simulink model "EPT"  (R2019b)
settings: Solver=FixedStepDiscrete  StartTime=0.0  StopTime=5  FixedStep=0.005  RelTol=1e-3  EnableMultiTasking=on
PreLoadFcn:
  | try, model_open; catch, disp('Error occurred while executing model pre-load callback: model_open.m'); disp('Please assure that the MATLAB working directory is set to the model directory before opening.'); end
InitFcn:
  | try, model_open; catch, end
undefined symbols (not defined in the file or in its folder): Bridge, GCM, H, ln, raptor_get_param_eval, raptor_get_safe_string, raptor_xcp_function
libraries: Raptor_lib x2810, simulink x374, hdlsllib x19
(part 4 of 45)

== system EPT/Foreground_TimeBase_5ms/CHG//DCHG_PW_Control/Maximum allowable torque ==
  note: P(KW)= Torque*rpm/9549.297
  Idchg_con : Inport
  Abs : Abs
  Abs1 : Abs
  Compare To Constant : simulink/Logic and Bit Operations/Compare To Constant  relop=<=  const=5  OutDataTypeStr=boolean
  Constant : Constant
  Data Type Conversion : DataTypeConversion
  Data Type Conversion1 : DataTypeConversion
  Data Type Conversion2 : DataTypeConversion
  Delay : Delay  DelayLength=1  InitialCondition=0
  Divide : Product  Inputs=*/
  Gain1 : Gain  Gain=0.01
  Gain2 : Gain  Gain=9.54805
  Min : MinMax  Inputs=2
  Product : Product  Inputs=3
  Product1 : Product
  Saturation : Saturate  UpperLimit=150  LowerLimit=0
  Saturation Dynamic1 : simulink/Discontinuities/Saturation Dynamic  OutMin=[]  OutMax=[]  OutDataTypeStr=Inherit: Same as second input  OutDataType=fixdt(1, 16)  OutScaling=2^-10  DoSatur=off
  Subtract : Sum  Inputs=+-
  Switch : Switch  Criteria=u2 > Threshold
  raptor_adjustment1 : Raptor_lib/Data Storage/raptor_adjustment  paramName='Cal_Eff_Min'  nameSource=Parameter  initValue=0  dataType=double  storage=Calibration  calDispType=Number  calEnum={'False', 'True'}  calGain=1.0  calOffset=0.0  calMax=inf  calMin=-inf  calFormat='-1'  calUnit=''  calHelp=''  calAccess=1  calFunction=raptor_xcp_function(gcb)  calDispHeaders=off  calColHeaders={'Col1' 'Col2' 'Col3'}  calRowHeaders={'Row1' 'Row2' 'Row3'}
      settings: SourceProductName=Raptor
  raptor_adjustment2 : Raptor_lib/Data Storage/raptor_adjustment  paramName='Vehicle_system_power'  nameSource=Parameter  initValue=5000  dataType=double  storage=Calibration  calDispType=Number  calEnum={'False', 'True'}  calGain=1.0  calOffset=0.0  calMax=inf  calMin=-inf  calFormat='-1'  calUnit=''  calHelp=''  calAccess=1  calFunction=raptor_xcp_function(gcb)  calDispHeaders=off  calColHeaders={'Col1' 'Col2' 'Col3'}  calRowHeaders={'Row1' 'Row2' 'Row3'}
      settings: SourceProductName=Raptor
  raptor_adjustment3 : Raptor_lib/Data Storage/raptor_adjustment  paramName='Cal_Eff_Max'  nameSource=Parameter  initValue=100  dataType=double  storage=Calibration  calDispType=Number  calEnum={'False', 'True'}  calGain=1.0  calOffset=0.0  calMax=inf  calMin=-inf  calFormat='-1'  calUnit=''  calHelp=''  calAccess=1  calFunction=raptor_xcp_function(gcb)  calDispHeaders=off  calColHeaders={'Col1' 'Col2' 'Col3'}  calRowHeaders={'Row1' 'Row2' 'Row3'}
      settings: SourceProductName=Raptor
  raptor_data_read1 : Raptor_lib/Data Storage/raptor_data_read  dataName='EPT_BPOBU_VOLT'  dataShape=Scalar  idxSource=Input  idxRow=1  idxCol=1
      settings: SourceProductName=Raptor
  raptor_data_read2 : Raptor_lib/Data Storage/raptor_data_read  dataName='Read_Motor_Speed'  dataShape=Scalar  idxSource=Input  idxRow=1  idxCol=1
      settings: SourceProductName=Raptor
  raptor_data_read3 : Raptor_lib/Data Storage/raptor_data_read  dataName='Read_Motor_Temp'  dataShape=Scalar  idxSource=Input  idxRow=1  idxCol=1
      settings: SourceProductName=Raptor
  raptor_data_read4 : Raptor_lib/Data Storage/raptor_data_read  dataName='Read_Controller_Temp'  dataShape=Scalar  idxSource=Input  idxRow=1  idxCol=1
      settings: SourceProductName=Raptor
  raptor_data_write : Raptor_lib/Data Storage/raptor_data_write  dataName='EPT_MAX_DRV_TRQ'  dataShape=Scalar  idxSource=Input Port  idxRow=1  idxCol=1
      settings: SourceProductName=Raptor
  raptor_measurement1 : Raptor_lib/Data Storage/raptor_measurement  paramName='efficiency'  nameSource=Parameter  calDispType=Number  calEnum={'False', 'True'}  calGain=1.0  calOffset=0.0  calMax=inf  calMin=-inf  calFormat='-1'  calUnit=''  calHelp=''  calAccess=1  calFunction=raptor_xcp_function(gcb)  calVisible=on
      settings: SourceProductName=Raptor
  raptor_measurement3 : Raptor_lib/Data Storage/raptor_measurement  paramName='tqMax_con'  nameSource=Parameter  calDispType=Number  calEnum={'False', 'True'}  calGain=1.0  calOffset=0.0  calMax=inf  calMin=-inf  calFormat='-1'  calUnit=''  calHelp=''  calAccess=1  calFunction=raptor_xcp_function(gcb)  calVisible=on
      settings: SourceProductName=Raptor
  raptor_table_1d1 : Raptor_lib/Table Lookup/raptor_table_1d  dataName='Tcontroller2MaxTq_Ft'  initValue=[1 1 0]  dataType=double  storage=Calibration  initValueX=[0 60 80]  dataTypeXY=double  storageXY=Calibration  calVisible=on  showTable=on  calGain=1.0  calOffset=0.0  calMax=Inf  calMin=-Inf  calFormat='-1'  calUnit=''  calHelp=''  showBreakpoint=on  dataNameX=[]  calGainX=1.0  calOffsetX=0.0  calMaxX=Inf  calMinX=-Inf  calFormatX='-1'  calUnitX=''  calHelpX=''  calAccess=1  calFunction=raptor_xcp_function(gcb)  measureEnable=off  mName=[raptor_get_param_eval(gcb,'dataName'), '_Output']
      settings: SourceProductName=Raptor
  raptor_table_1d2 : Raptor_lib/Table Lookup/raptor_table_1d  dataName='Tmotor2MaxTq_Ft'  initValue=[1 1 0]  dataType=double  storage=Calibration  initValueX=[0 100 120]  dataTypeXY=double  storageXY=Calibration  calVisible=on  showTable=on  calGain=1.0  calOffset=0.0  calMax=Inf  calMin=-Inf  calFormat='-1'  calUnit=''  calHelp=''  showBreakpoint=on  dataNameX=[]  calGainX=1.0  calOffsetX=0.0  calMaxX=Inf  calMinX=-Inf  calFormatX='-1'  calUnitX=''  calHelpX=''  calAccess=1  calFunction=raptor_xcp_function(gcb)  measureEnable=off  mName=[raptor_get_param_eval(gcb,'dataName'), '_Output']
      settings: SourceProductName=Raptor
  raptor_table_2d : Raptor_lib/Table Lookup/raptor_table_2d  dataName='Efficiency'  initValue=|  dataType=double  storage=Calibration  initValueX="[0\t300\t600\t1200\t1800\t2400\t3000\t3600\t4200\t4800\t5400\t6000]"  initValueY="[0\t7.5\t15\t30\t45\t60\t75\t90\t105\t120\t135\t150]"  dataTypeXY=double  storageXY=Calibration  calVisible=on  showTable=off  calGain=1.0  calOffset=0.0  calMax=Inf  calMin=-Inf  calFormat='-1'  calUnit=''  calHelp=''  showBreakpointX=off  dataNameX=[]  calGainX=1.0  calOffsetX=0.0  calMaxX=Inf  calMinX=-Inf  calFormatX='-1'  calUnitX=''  calHelpX=''  showBreakpointY=off  dataNameY=[]  calGainY=1.0  calOffsetY=0.0  calMaxY=Inf  calMinY=-Inf  calFormatY='-1'  calUnitY=''  calHelpY=''  calAccess=1  calFunction=raptor_xcp_function(gcb)  measureEnable=off  mName=[raptor_get_param_eval(gcb,'dataName'), '_Output']
      | [50	50	50	50	50	50	50	50	50	50	50	50;
      | 55	60	62.5	65	70	72.5	75	77.5	77.5	75	72.5	70;
      | 57.5	62.5	65	70	77.5	80	80	82.5	82.5	80	77.5	75;
      | 57.5	65	67.5	72.5	80	82.5	85	85	85	85	85	82.5;
      | 60	67.5	70	80	85	85	87.5	87.5	87.5	87.5	87.5	85;
      | 60	67.5	72.5	82.5	87.5	87.5	90	90	90	87.5	85	82.5;
      | 62.5	70	75	82.5	87.5	90	90	87.5	85	82.5	82.5	80;
      | 62.5	72.5	77.5	85	90	90	87.5	85	82.5	80	80	77.5;
      | 65	72.5	77.5	85	90	90	85	82.5	80	77.5	80	75;
      | 65	72.5	75	82.5	90	87.5	82.5	80	80	75	77.5	72.5;
      | 67.5	70	75	82.5	87.5	85	82.5	80	77.5	75	75	70;
      | 67.5	70	72.5	80	85	82.5	77.5	75	77.5	72.5	75	70;]
      settings: SourceProductName=Raptor
  wires:
  Gain2/1 -> Divide/1
  Idchg_con/1 -> Abs/1
  Subtract/1 -> Gain2/1
  raptor_adjustment2/1 -> Subtract/2
  Switch/1 -> Divide/2
  Product/1 -> Subtract/1
  Abs/1 -> Product/3
  raptor_data_read1/1 -> Product/2
  raptor_data_read2/1 -> Abs1/1
  Compare To Constant/1 -> Switch/2
  Constant/1 -> Switch/1
  Saturation Dynamic1/1 -> raptor_measurement1/1, Gain1/1
  Gain1/1 -> Product/1
  Abs1/1 -> Data Type Conversion/1
  Data Type Conversion/1 -> raptor_table_2d/2, Switch/3, Compare To Constant/1
  Divide/1 -> Saturation/1
  Delay/1 -> raptor_table_2d/1
  Data Type Conversion1/1 -> raptor_data_write/1
  raptor_data_read3/1 -> raptor_table_1d2/1
  Min/1 -> Product1/1
  Saturation/1 -> Product1/2, Delay/1
  Product1/1 -> Data Type Conversion1/1, raptor_measurement3/1
  raptor_table_2d/1 -> Saturation Dynamic1/2
  raptor_adjustment3/1 -> Saturation Dynamic1/1
  raptor_adjustment1/1 -> Saturation Dynamic1/3
  raptor_data_read4/1 -> Data Type Conversion2/1
  raptor_table_1d1/1 -> Min/1
  raptor_table_1d2/1 -> Min/2
  Data Type Conversion2/1 -> raptor_table_1d1/1

== system EPT/Foreground_TimeBase_5ms/CHG//DCHG_PW_Control/PWCU PW Requirement ==

== system EPT/Foreground_TimeBase_5ms/CHG//DCHG_PW_Control/SWU Power Divider ==
  PWCU : Subsystem

== system EPT/Foreground_TimeBase_5ms/Delay/CycleTrigger ==
  In1 : Inport
  In2 : Inport  Port=2
  Add : Sum
  Add1 : Sum
  Add2 : Sum  Inputs=+-
  Constant1 : Constant
  Constant2 : Constant  Value=0
  Constant3 : Constant
  Data Type Conversion1 : DataTypeConversion
  Data Type Conversion2 : DataTypeConversion
  Display : Display
  Relational Operator1 : RelationalOperator  OutDataTypeStr=boolean  RndMeth=Simplest
  Saturation : Saturate  UpperLimit=inf  LowerLimit=2
  Scope : Scope
  Scope1 : Scope
  Scope2 : Scope
  Switch : Switch  Threshold=1
  Unit Delay : UnitDelay  SampleTime=-1  HasFrameUpgradeWarning=on
  Unit Delay1 : UnitDelay  SampleTime=-1  HasFrameUpgradeWarning=on
  Trigger : Outport  VectorParamsAs1DForOutWhenUnconnected=off
  wires:
  Saturation/1 -> Add2/1
  Add/1 -> Switch/1
  In1/1 -> Data Type Conversion2/1
  Unit Delay/1 -> Add/1
  Switch/1 -> Relational Operator1/1, Scope1/1, Unit Delay/1
  Add1/1 -> Scope/1, Unit Delay1/1, Display/1
  Unit Delay1/1 -> Add1/1
  Constant1/1 -> Add1/2
  Relational Operator1/1 -> Scope2/1, Trigger/1
  Data Type Conversion1/1 -> Relational Operator1/2
  Constant2/1 -> Switch/3
  Data Type Conversion2/1 -> Add/2, Switch/2
  Add2/1 -> Data Type Conversion1/1
  In2/1 -> Saturation/1
  Constant3/1 -> Add2/2

== system EPT/Foreground_TimeBase_5ms/E//W /BP-OBU_E//W ==
  BP-OBU_E/W : Subsystem
  Delay : Subsystem
  Latch : Subsystem
  Logical Operator1 : Logic  Inputs=3  AllPortsSameDT=off  OutDataTypeStr=boolean
  NOT : Logic  Operator=NOT  IconShape=distinctive  AllPortsSameDT=off  OutDataTypeStr=boolean
  NOT1 : Logic  Operator=NOT  IconShape=distinctive  AllPortsSameDT=off  OutDataTypeStr=boolean
  NOT2 : Logic  Operator=NOT  IconShape=distinctive  AllPortsSameDT=off  OutDataTypeStr=boolean
  raptor_adjustment : Raptor_lib/Data Storage/raptor_adjustment  paramName='Cal_BPOBU_EW_Check_TimeCount'  nameSource=Parameter  initValue=400  dataType=double  storage=Calibration  calDispType=Number  calEnum={'False', 'True'}  calGain=1.0  calOffset=0.0  calMax=inf  calMin=-inf  calFormat='-1'  calUnit=''  calHelp=''  calAccess=1  calFunction=raptor_xcp_function(gcb)  calDispHeaders=off  calColHeaders={'Col1' 'Col2' 'Col3'}  calRowHeaders={'Row1' 'Row2' 'Row3'}
      settings: SourceProductName=Raptor
  raptor_data_read1 : Raptor_lib/Data Storage/raptor_data_read  dataName='CMU_Ready'  dataShape=Scalar  idxSource=Input  idxRow=1  idxCol=1
      settings: SourceProductName=Raptor
  raptor_data_read19 : Raptor_lib/Data Storage/raptor_data_read  dataName='CAN_Fault_CMU1'  dataShape=Scalar  idxSource=Input  idxRow=1  idxCol=1
      settings: SourceProductName=Raptor
  raptor_data_read20 : Raptor_lib/Data Storage/raptor_data_read  dataName='CAN_Fault_CMU2'  dataShape=Scalar  idxSource=Input  idxRow=1  idxCol=1
      settings: SourceProductName=Raptor
  wires:
  Delay/1(Output) -> Latch/1(Latch)
  raptor_data_read19/1 -> NOT/1
  raptor_data_read20/1 -> NOT1/1
  raptor_adjustment/1 -> Delay/2(TimeCount)
  Logical Operator1/1 -> NOT2/1, Delay/1(Condition)
  NOT/1 -> Logical Operator1/2
  NOT2/1 -> Latch/2(Reset)
  NOT1/1 -> Logical Operator1/3
  Latch/1(Output) -> BP-OBU_E/W/1("CMU_Work ")
  raptor_data_read1/1 -> Logical Operator1/1

== system EPT/Foreground_TimeBase_5ms/E//W /CAN_E//W ==
  CAN_Abnormal : Subsystem
  CAN_Fault : Subsystem

== system EPT/Foreground_TimeBase_5ms/E//W /E//W_Process ==
  CAN_Fault : Subsystem
  Data Type Conversion1 : DataTypeConversion
  ECHS_Fault : Subsystem
  Logical Operator : Logic  Operator=OR  Inputs=6  AllPortsSameDT=off  OutDataTypeStr=boolean
  OBU_Fault : Subsystem
  Switch3 : Switch  Threshold=1
  raptor_adjustment1 : Raptor_lib/Data Storage/raptor_adjustment  paramName='Cal_Alarm_Manual'  nameSource=Parameter  initValue=0.00  dataType=boolean  storage=Calibration  calDispType=Number  calEnum={'False', 'True'}  calGain=1.0  calOffset=0.0  calMax=inf  calMin=-inf  calFormat='-1'  calUnit=''  calHelp=''  calAccess=1  calFunction=raptor_xcp_function(gcb)  calDispHeaders=off  calColHeaders={'Col1' 'Col2' 'Col3'}  calRowHeaders={'Row1' 'Row2' 'Row3'}
      settings: SourceProductName=Raptor
  raptor_adjustment2 : Raptor_lib/Data Storage/raptor_adjustment  paramName='Cal_Alarm_Manual_EN'  nameSource=Parameter  initValue=0.00  dataType=boolean  storage=Calibration  calDispType=Number  calEnum={'False', 'True'}  calGain=1.0  calOffset=0.0  calMax=inf  calMin=-inf  calFormat='-1'  calUnit=''  calHelp=''  calAccess=1  calFunction=raptor_xcp_function(gcb)  calDispHeaders=off  calColHeaders={'Col1' 'Col2' 'Col3'}  calRowHeaders={'Row1' 'Row2' 'Row3'}
      settings: SourceProductName=Raptor
  raptor_data_def6 : Raptor_lib/Data Storage/raptor_data_def  dataName='EPT_EW_STA'  initValue=0  dataType=boolean  storage=Volatile (RAM)  calVisible=on  calType=Measurement  calDispType=Number  calEnum={'False', 'True'}  calGain=1.0  calOffset=0  calMin=-inf  calMax=inf  calFormat='-1'  calUnit=''  calHelp=''  calAccess=1  calFunction=raptor_xcp_function(gcb)  calDispHeaders=off  calColHeaders={'Col1' 'Col2' 'Col3'}  calRowHeaders={'Row1' 'Row2' 'Row3'}
      settings: SourceProductName=Raptor
  raptor_data_write4 : Raptor_lib/Data Storage/raptor_data_write  dataName='EPT_EW_STA'  dataShape=Scalar  idxSource=Input Port  idxRow=1  idxCol=1
      settings: SourceProductName=Raptor
  wires:
  raptor_adjustment2/1 -> Switch3/2
  Switch3/1 -> Data Type Conversion1/1
  raptor_adjustment1/1 -> Switch3/1
  Data Type Conversion1/1 -> raptor_data_write4/1
  CAN_Fault/1(Fault) -> Logical Operator/1
  Logical Operator/1 -> Switch3/3
  ECHS_Fault/1(Fault) -> Logical Operator/2
  OBU_Fault/1(G1_Fault) -> Logical Operator/3
  OBU_Fault/2(G2_Fault) -> Logical Operator/4
  OBU_Fault/3(G3_Fault) -> Logical Operator/5
  OBU_Fault/4(G4_Fault) -> Logical Operator/6

== system EPT/Foreground_TimeBase_5ms/OBP_Temp_Detection/ADC2Degree ==
  Trigger : TriggerPort  VariantControl=Variant  PortDimensions=1
  Data Type Conversion : DataTypeConversion
  Demux : Demux
  Gain : Gain  Gain=1/4
  MinMax : MinMax  Function=max
  MinMax1 : MinMax
  Mux : Mux
  Mux1 : Mux
  Sum of Elements : Sum  Inputs=+
  raptor_data_def1 : Raptor_lib/Data Storage/raptor_data_def  dataName='Temp_1'  initValue=0  dataType=double  storage=Volatile (RAM)  calVisible=on  calType=Measurement  calDispType=Number  calEnum={'False', 'True'}  calGain=1.0  calOffset=0  calMin=-inf  calMax=inf  calFormat='-1'  calUnit=''  calHelp=''  calAccess=1  calFunction=raptor_xcp_function(gcb)  calDispHeaders=off  calColHeaders={'Col1' 'Col2' 'Col3'}  calRowHeaders={'Row1' 'Row2' 'Row3'}
      settings: SourceProductName=Raptor
  raptor_data_def2 : Raptor_lib/Data Storage/raptor_data_def  dataName='Temp_2'  initValue=0  dataType=double  storage=Volatile (RAM)  calVisible=on  calType=Measurement  calDispType=Number  calEnum={'False', 'True'}  calGain=1.0  calOffset=0  calMin=-inf  calMax=inf  calFormat='-1'  calUnit=''  calHelp=''  calAccess=1  calFunction=raptor_xcp_function(gcb)  calDispHeaders=off  calColHeaders={'Col1' 'Col2' 'Col3'}  calRowHeaders={'Row1' 'Row2' 'Row3'}
      settings: SourceProductName=Raptor
  raptor_data_def3 : Raptor_lib/Data Storage/raptor_data_def  dataName='Temp_3'  initValue=0  dataType=double  storage=Volatile (RAM)  calVisible=on  calType=Measurement  calDispType=Number  calEnum={'False', 'True'}  calGain=1.0  calOffset=0  calMin=-inf  calMax=inf  calFormat='-1'  calUnit=''  calHelp=''  calAccess=1  calFunction=raptor_xcp_function(gcb)  calDispHeaders=off  calColHeaders={'Col1' 'Col2' 'Col3'}  calRowHeaders={'Row1' 'Row2' 'Row3'}
      settings: SourceProductName=Raptor
  raptor_data_def4 : Raptor_lib/Data Storage/raptor_data_def  dataName='Temp_4'  initValue=0  dataType=double  storage=Volatile (RAM)  calVisible=on  calType=Measurement  calDispType=Number  calEnum={'False', 'True'}  calGain=1.0  calOffset=0  calMin=-inf  calMax=inf  calFormat='-1'  calUnit=''  calHelp=''  calAccess=1  calFunction=raptor_xcp_function(gcb)  calDispHeaders=off  calColHeaders={'Col1' 'Col2' 'Col3'}  calRowHeaders={'Row1' 'Row2' 'Row3'}
      settings: SourceProductName=Raptor
  raptor_data_def5 : Raptor_lib/Data Storage/raptor_data_def  dataName='BP_OBU_Tbp_Down'  initValue=0  dataType=double  storage=Volatile (RAM)  calVisible=on  calType=Measurement  calDispType=Number  calEnum={'False', 'True'}  calGain=1.0  calOffset=0  calMin=-inf  calMax=inf  calFormat='-1'  calUnit=''  calHelp=''  calAccess=1  calFunction=raptor_xcp_function(gcb)  calDispHeaders=off  calColHeaders={'Col1' 'Col2' 'Col3'}  calRowHeaders={'Row1' 'Row2' 'Row3'}
      settings: SourceProductName=Raptor
  raptor_data_def6 : Raptor_lib/Data Storage/raptor_data_def  dataName='BP_OBU_Tbp_Up'  initValue=0  dataType=double  storage=Volatile (RAM)  calVisible=on  calType=Measurement  calDispType=Number  calEnum={'False', 'True'}  calGain=1.0  calOffset=0  calMin=-inf  calMax=inf  calFormat='-1'  calUnit=''  calHelp=''  calAccess=1  calFunction=raptor_xcp_function(gcb)  calDispHeaders=off  calColHeaders={'Col1' 'Col2' 'Col3'}  calRowHeaders={'Row1' 'Row2' 'Row3'}
      settings: SourceProductName=Raptor
  raptor_data_def7 : Raptor_lib/Data Storage/raptor_data_def  dataName='BP_OBU_Tair_In'  initValue=0  dataType=double  storage=Volatile (RAM)  calVisible=on  calType=Measurement  calDispType=Number  calEnum={'False', 'True'}  calGain=1.0  calOffset=0  calMin=-inf  calMax=inf  calFormat='-1'  calUnit=''  calHelp=''  calAccess=1  calFunction=raptor_xcp_function(gcb)  calDispHeaders=off  calColHeaders={'Col1' 'Col2' 'Col3'}  calRowHeaders={'Row1' 'Row2' 'Row3'}
      settings: SourceProductName=Raptor
  raptor_data_def8 : Raptor_lib/Data Storage/raptor_data_def  dataName='BP_OBU_Tair_Out'  initValue=0  dataType=double  storage=Volatile (RAM)  calVisible=on  calType=Measurement  calDispType=Number  calEnum={'False', 'True'}  calGain=1.0  calOffset=0  calMin=-inf  calMax=inf  calFormat='-1'  calUnit=''  calHelp=''  calAccess=1  calFunction=raptor_xcp_function(gcb)  calDispHeaders=off  calColHeaders={'Col1' 'Col2' 'Col3'}  calRowHeaders={'Row1' 'Row2' 'Row3'}
      settings: SourceProductName=Raptor
  raptor_data_def9 : Raptor_lib/Data Storage/raptor_data_def  dataName='BP_OBU_Tair_Avarage'  initValue=0  dataType=double  storage=Volatile (RAM)  calVisible=on  calType=Measurement  calDispType=Number  calEnum={'False', 'True'}  calGain=1.0  calOffset=0  calMin=-inf  calMax=inf  calFormat='-1'  calUnit=''  calHelp=''  calAccess=1  calFunction=raptor_xcp_function(gcb)  calDispHeaders=off  calColHeaders={'Col1' 'Col2' 'Col3'}  calRowHeaders={'Row1' 'Row2' 'Row3'}
      settings: SourceProductName=Raptor
  raptor_data_read5 : Raptor_lib/Data Storage/raptor_data_read  dataName='TBP_2'  dataShape=Scalar  idxSource=Input  idxRow=1  idxCol=1
      settings: SourceProductName=Raptor
  raptor_data_read6 : Raptor_lib/Data Storage/raptor_data_read  dataName='TBP_3'  dataShape=Scalar  idxSource=Input  idxRow=1  idxCol=1
      settings: SourceProductName=Raptor
  raptor_data_read7 : Raptor_lib/Data Storage/raptor_data_read  dataName='TBP_4'  dataShape=Scalar  idxSource=Input  idxRow=1  idxCol=1
      settings: SourceProductName=Raptor
  raptor_data_read8 : Raptor_lib/Data Storage/raptor_data_read  dataName='TBP_1'  dataShape=Scalar  idxSource=Input  idxRow=1  idxCol=1
      settings: SourceProductName=Raptor
  raptor_data_write1 : Raptor_lib/Data Storage/raptor_data_write  dataName='BP_OBU_Tbp_Up'  dataShape=Scalar  idxSource=Input Port  idxRow=1  idxCol=1
      settings: SourceProductName=Raptor
  raptor_data_write2 : Raptor_lib/Data Storage/raptor_data_write  dataName='BP_OBU_Tbp_Down'  dataShape=Scalar  idxSource=Input Port  idxRow=1  idxCol=1
      settings: SourceProductName=Raptor
  raptor_data_write3 : Raptor_lib/Data Storage/raptor_data_write  dataName='BP_OBU_Tair_Out'  dataShape=Scalar  idxSource=Input Port  idxRow=1  idxCol=1
      settings: SourceProductName=Raptor
  raptor_data_write4 : Raptor_lib/Data Storage/raptor_data_write  dataName='Temp_1'  dataShape=Scalar  idxSource=Input Port  idxRow=1  idxCol=1
      settings: SourceProductName=Raptor
  raptor_data_write5 : Raptor_lib/Data Storage/raptor_data_write  dataName='Temp_2'  dataShape=Scalar  idxSource=Input Port  idxRow=1  idxCol=1
      settings: SourceProductName=Raptor
  raptor_data_write6 : Raptor_lib/Data Storage/raptor_data_write  dataName='Temp_3'  dataShape=Scalar  idxSource=Input Port  idxRow=1  idxCol=1
      settings: SourceProductName=Raptor
  raptor_data_write7 : Raptor_lib/Data Storage/raptor_data_write  dataName='Temp_4'  dataShape=Scalar  idxSource=Input Port  idxRow=1  idxCol=1
      settings: SourceProductName=Raptor
  raptor_data_write8 : Raptor_lib/Data Storage/raptor_data_write  dataName='BP_OBU_Tair_In'  dataShape=Scalar  idxSource=Input Port  idxRow=1  idxCol=1
      settings: SourceProductName=Raptor
  raptor_data_write9 : Raptor_lib/Data Storage/raptor_data_write  dataName='BP_OBU_Tair_Avarage'  dataShape=Scalar  idxSource=Input Port  idxRow=1  idxCol=1
      settings: SourceProductName=Raptor
  raptor_table_1d1 : Raptor_lib/Table Lookup/raptor_table_1d  dataName='ADC2Degree'  initValue="[-20\t-19\t-18\t-17\t-16\t-15\t-14\t-13\t-12\t-11\t-10\t-9\t-8\t-7\t-6\t-5\t-4\t-3\t-2\t-1\t0\t1\t2\t3\t4\t5\t6\t7\t8\t9\t10\t11\t12\t13\t14\t15\t16\t17\t18\t19\t20\t21\t22\t23\t24\t25\t26\t27\t28\t29\t30\t31\t32\t33\t34\t35\t36\t37\t38\t39\t40\t41\t42\t43\t44\t45\t46\t47\t48\t49\t50\t51\t52\t53\t54\t55\t56\t57\t58\t59\t60\t61\t62\t63\t64\t65\t66\t67\t68\t69\t70\t71\t72\t73\t74\t75\t76\t77\t78\t79\t80\t81\t82\t83\t84\t85\t86\t87\t88\t89\t90\t91\t92\t93\t94\t95\t96\t97\t98\t99\t100]"  dataType=double  storage=Calibration  initValueX="[3970.851347\t3964.877034\t3958.660648\t3952.19673\t3945.478916\t3938.499476\t3931.248745\t3923.724418\t3915.91351\t3907.814925\t3899.415195\t3890.710838\t3881.692913\t3872.355604\t3862.69176\t3852.692308\t3842.352789\t3831.667763\t3820.621728\t3809.221955\t3797.448545\t3785.307433\t3772.783267\t3759.880862\t3746.57901\t3732.878913\t3718.782155\t3704.273066\t3689.367657\t3674.026011\t3658.28125\t3642.106481\t3625.515118\t3608.469828\t3591.007213\t3573.112033\t3554.79568\t3536.03549\t3516.838061\t3497.210076\t3477.157895\t3456.640806\t3435.70316\t3414.346734\t3392.570608\t3370.37037\t3347.673797\t3324.657013\t3301.252254\t3277.369056\t3253.13253\t3228.439961\t3203.43038\t3178.08165\t3152.259878\t3126.11588\t3099.607123\t3072.795193\t3045.625745\t3018.159247\t2990.326223\t2962.329217\t2933.948965\t2905.236486\t2876.418685\t2847.232143\t2817.911227\t2788.343722\t2758.592896\t2728.72905\t2698.386739\t2668.286339\t2637.825223\t2607.293004\t2576.502242\t2545.774239\t2514.91206\t2483.975297\t2453.028721\t2422.142314\t2391.061544\t2359.830508\t2328.851555\t2297.84752\t2266.875\t2235.99451\t2205.270444\t2174.770992\t2144.13583\t2113.39973\t2083.059872\t2052.724426\t2022.436441\t1992.743553\t1962.704045\t1933.386938\t1903.797909\t1874.508197\t1845.574859\t1817.056921\t1788.411056\t1760.274463\t1732.077295\t1703.840304\t1676.914309\t1649.375\t1622.590564\t1595.922509\t1569.39759\t1543.043478\t1516.888726\t1491.732703\t1466.08092\t1441.518987\t1416.493763\t1392.651934\t1368.381852\t1344.531396\t1321.134216\t1298.224269\t1275.835735]"  dataTypeXY=double  storageXY=Calibration  calVisible=on  showTable=on  calGain=1.0  calOffset=0.0  calMax=Inf  calMin=-Inf  calFormat='-1'  calUnit=''  calHelp=''  showBreakpoint=on  dataNameX=[]  calGainX=1.0  calOffsetX=0.0  calMaxX=Inf  calMinX=-Inf  calFormatX='-1'  calUnitX=''  calHelpX=''  calAccess=1  calFunction=raptor_xcp_function(gcb)  measureEnable=off  mName=[raptor_get_param_eval(gcb,'dataName'), '_Output']
      settings: SourceProductName=Raptor
  wires:
  Demux/3 -> raptor_data_write6/1, raptor_data_write3/1, Mux1/2
  raptor_table_1d1/1 -> Sum of Elements/1, Demux/1
  Mux/1 -> Data Type Conversion/1
  raptor_data_read8/1 -> Mux/1
  raptor_data_read6/1 -> Mux/3
  raptor_data_read7/1 -> Mux/4
  raptor_data_read5/1 -> Mux/2
  Data Type Conversion/1 -> raptor_table_1d1/1
  Mux1/1 -> MinMax1/1, MinMax/1
  Demux/1 -> Mux1/4, raptor_data_write4/1
  Demux/4 -> Mux1/1, raptor_data_write7/1
  MinMax/1 -> raptor_data_write1/1
  MinMax1/1 -> raptor_data_write2/1
  Demux/2 -> Mux1/3, raptor_data_write5/1, raptor_data_write8/1
  Sum of Elements/1 -> Gain/1
  Gain/1 -> raptor_data_write9/1

== system EPT/Foreground_TimeBase_5ms/OBP_Temp_Detection/CountTrigger ==
  Counter : Inport
  Constant1 : Constant  Value=0
  Constant3 : Constant
  CycleTrigger : Subsystem
  Switch : Switch  Threshold=1
  Unit Delay1 : UnitDelay  SampleTime=-1  HasFrameUpgradeWarning=on
  Unit Delay2 : UnitDelay  SampleTime=-1  HasFrameUpgradeWarning=on
  Tirgger : Outport  VectorParamsAs1DForOutWhenUnconnected=off
  wires:
  Switch/1 -> Unit Delay1/1
  Constant3/1 -> Switch/3
  Constant1/1 -> Switch/1
  Counter/1 -> CycleTrigger/2(In2)
  CycleTrigger/1(Trigger) -> Switch/2, Unit Delay2/1
  Unit Delay1/1 -> CycleTrigger/1(In1)
  Unit Delay2/1 -> Tirgger/1

== system EPT/Foreground_TimeBase_5ms/Oil//Water//Pack Cooling System/AirC ==
  MaxTcell : Inport
  PW : Inport  Port=2
  Constant : Constant  Value=100
  Product3 : Product
  Saturation Dynamic2 : simulink/Discontinuities/Saturation Dynamic  OutMin=[]  OutMax=[]  OutDataTypeStr=Inherit: Same as second input  OutDataType=fixdt(1, 16)  OutScaling=2^-10  DoSatur=off
  raptor_adjustment4 : Raptor_lib/Data Storage/raptor_adjustment  paramName='Cal_BlowerIdleDuty_Low_Saturation'  nameSource=Parameter  initValue=60  dataType=double  storage=Calibration  calDispType=Number  calEnum={'False', 'True'}  calGain=1.0  calOffset=0.0  calMax=inf  calMin=-inf  calFormat='-1'  calUnit=''  calHelp=''  calAccess=1  calFunction=raptor_xcp_function(gcb)  calDispHeaders=off  calColHeaders={'Col1' 'Col2' 'Col3'}  calRowHeaders={'Row1' 'Row2' 'Row3'}
      settings: SourceProductName=Raptor
  raptor_table_1d4 : Raptor_lib/Table Lookup/raptor_table_1d  dataName='Tcell2BlowerDutyFt'  initValue=[0.5,1,1,10,10]  dataType=double  storage=Calibration  initValueX=[0,35,40,45,55]  dataTypeXY=double  storageXY=Calibration  calVisible=on  showTable=on  calGain=1.0  calOffset=0.0  calMax=Inf  calMin=-Inf  calFormat='-1'  calUnit=''  calHelp=''  showBreakpoint=on  dataNameX=[]  calGainX=1.0  calOffsetX=0.0  calMaxX=Inf  calMinX=-Inf  calFormatX='-1'  calUnitX=''  calHelpX=''  calAccess=1  calFunction=raptor_xcp_function(gcb)  measureEnable=off  mName=[raptor_get_param_eval(gcb,'dataName'), '_Output']
      settings: SourceProductName=Raptor
  Duty : Outport
  wires:
  PW/1 -> Product3/2
  raptor_adjustment4/1 -> Saturation Dynamic2/3
  raptor_table_1d4/1 -> Product3/1
  Constant/1 -> Saturation Dynamic2/1
  MaxTcell/1 -> raptor_table_1d4/1
  Saturation Dynamic2/1 -> Duty/1
  Product3/1 -> Saturation Dynamic2/2

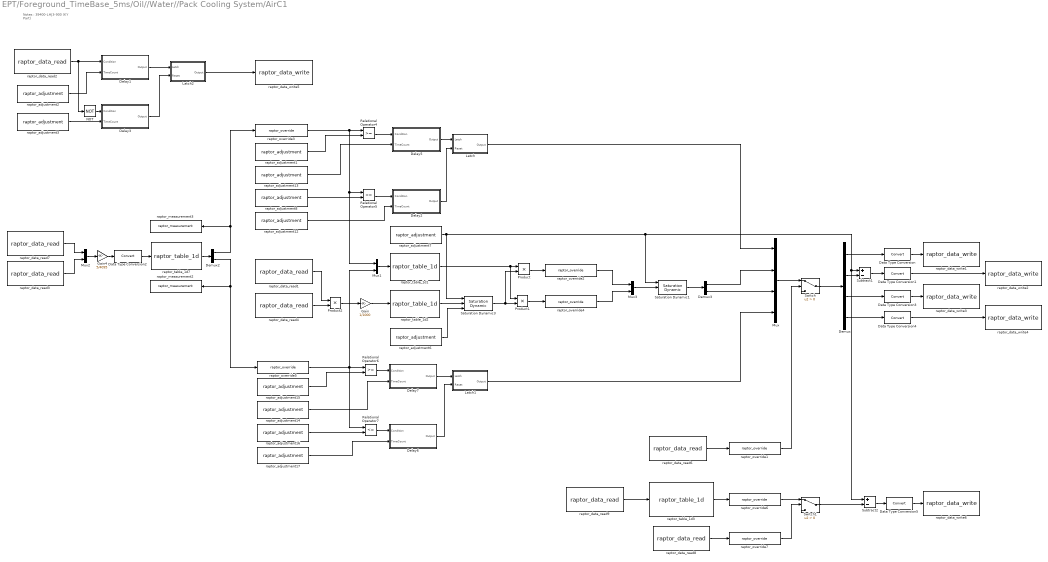
== system EPT/Foreground_TimeBase_5ms/Oil//Water//Pack Cooling System/AirC1 ==
  note: Notes :
      | 39400-LHJ3-900
      | (KY Part)
  Data Type Conversion{,1..5} (6 alike) : DataTypeConversion
  Delay1 : Subsystem
  Delay2 : Subsystem
  Delay3 : Subsystem
  Delay5 : Subsystem
  Delay6 : Subsystem
  Delay7 : Subsystem
  Demux : Demux
  Demux2 : Demux  Outputs=2
  Demux3 : Demux  Outputs=2
  Gain : Gain  Gain=1/1000
  Gain4 : Gain  Gain=5/4095
  Latch : Subsystem
  Latch1 : Subsystem
  Latch2 : Subsystem
  Mux : Mux
  Mux1 : Mux  Inputs=2
  Mux2 : Mux  Inputs=2
  Mux3 : Mux  Inputs=2
  NOT : Logic  Operator=NOT  IconShape=distinctive  AllPortsSameDT=off  OutDataTypeStr=boolean
  Product : Product
  Product1 : Product
  Product2 : Product
  Relational Operator4 : RelationalOperator  OutDataTypeStr=boolean  RndMeth=Simplest
  Relational Operator5 : RelationalOperator  Operator=<=  OutDataTypeStr=boolean  RndMeth=Simplest
  Relational Operator6 : RelationalOperator  OutDataTypeStr=boolean  RndMeth=Simplest
  Relational Operator7 : RelationalOperator  Operator=<=  OutDataTypeStr=boolean  RndMeth=Simplest
  Saturation Dynamic1 : simulink/Discontinuities/Saturation Dynamic  OutMin=[]  OutMax=[]  OutDataTypeStr=Inherit: Same as second input  OutDataType=fixdt(1, 16)  OutScaling=2^-10  DoSatur=off
  Saturation Dynamic3 : simulink/Discontinuities/Saturation Dynamic  OutMin=[]  OutMax=[]  OutDataTypeStr=Inherit: Same as second input  OutDataType=fixdt(1, 16)  OutScaling=2^-10  DoSatur=off
  Subtract1 : Sum  Inputs=+-
  Subtract2 : Sum  Inputs=+-
  Switch : Switch  Criteria=u2 > Threshold
  Switch1 : Switch  Criteria=u2 > Threshold
  raptor_adjustment1 : Raptor_lib/Data Storage/raptor_adjustment  paramName='Cal_Cooling_Water_Temp_LimitHigh'  nameSource=Parameter  initValue=55  dataType=double  storage=Calibration  calDispType=Number  calEnum={'False', 'True'}  calGain=1.0  calOffset=0.0  calMax=inf  calMin=-inf  calFormat='-1'  calUnit=''  calHelp=''  calAccess=1  calFunction=raptor_xcp_function(gcb)  calDispHeaders=off  calColHeaders={'Col1' 'Col2' 'Col3'}  calRowHeaders={'Row1' 'Row2' 'Row3'}
      settings: SourceProductName=Raptor
  raptor_adjustment12 : Raptor_lib/Data Storage/raptor_adjustment  paramName='Cal_Water_Cooling_Fan_Off_DelayTime'  nameSource=Parameter  initValue=1000  dataType=double  storage=Calibration  calDispType=Number  calEnum={'False', 'True'}  calGain=1.0  calOffset=0.0  calMax=inf  calMin=-inf  calFormat='-1'  calUnit=''  calHelp=''  calAccess=1  calFunction=raptor_xcp_function(gcb)  calDispHeaders=off  calColHeaders={'Col1' 'Col2' 'Col3'}  calRowHeaders={'Row1' 'Row2' 'Row3'}
      settings: SourceProductName=Raptor
  raptor_adjustment13 : Raptor_lib/Data Storage/raptor_adjustment  paramName='Cal_Water_Cooling_Fan_On_DelayTime'  nameSource=Parameter  initValue=0.00  dataType=double  storage=Calibration  calDispType=Number  calEnum={'False', 'True'}  calGain=1.0  calOffset=0.0  calMax=inf  calMin=-inf  calFormat='-1'  calUnit=''  calHelp=''  calAccess=1  calFunction=raptor_xcp_function(gcb)  calDispHeaders=off  calColHeaders={'Col1' 'Col2' 'Col3'}  calRowHeaders={'Row1' 'Row2' 'Row3'}
      settings: SourceProductName=Raptor
  raptor_adjustment14 : Raptor_lib/Data Storage/raptor_adjustment  paramName='Cal_Oil_Cooling_Fan_On_DelayTime'  nameSource=Parameter  initValue=0.00  dataType=double  storage=Calibration  calDispType=Number  calEnum={'False', 'True'}  calGain=1.0  calOffset=0.0  calMax=inf  calMin=-inf  calFormat='-1'  calUnit=''  calHelp=''  calAccess=1  calFunction=raptor_xcp_function(gcb)  calDispHeaders=off  calColHeaders={'Col1' 'Col2' 'Col3'}  calRowHeaders={'Row1' 'Row2' 'Row3'}
      settings: SourceProductName=Raptor
  raptor_adjustment15 : Raptor_lib/Data Storage/raptor_adjustment  paramName='Cal_Cooling_Oil_Temp_LimitHigh'  nameSource=Parameter  initValue=70  dataType=double  storage=Calibration  calDispType=Number  calEnum={'False', 'True'}  calGain=1.0  calOffset=0.0  calMax=inf  calMin=-inf  calFormat='-1'  calUnit=''  calHelp=''  calAccess=1  calFunction=raptor_xcp_function(gcb)  calDispHeaders=off  calColHeaders={'Col1' 'Col2' 'Col3'}  calRowHeaders={'Row1' 'Row2' 'Row3'}
      settings: SourceProductName=Raptor
  raptor_adjustment16 : Raptor_lib/Data Storage/raptor_adjustment  paramName='Cal_Cooling_Oil_Temp_LimitLow'  nameSource=Parameter  initValue=60  dataType=double  storage=Calibration  calDispType=Number  calEnum={'False', 'True'}  calGain=1.0  calOffset=0.0  calMax=inf  calMin=-inf  calFormat='-1'  calUnit=''  calHelp=''  calAccess=1  calFunction=raptor_xcp_function(gcb)  calDispHeaders=off  calColHeaders={'Col1' 'Col2' 'Col3'}  calRowHeaders={'Row1' 'Row2' 'Row3'}
      settings: SourceProductName=Raptor
  raptor_adjustment17 : Raptor_lib/Data Storage/raptor_adjustment  paramName='Cal_Oil_Cooling_Fan_Off_DelayTime'  nameSource=Parameter  initValue=3000  dataType=double  storage=Calibration  calDispType=Number  calEnum={'False', 'True'}  calGain=1.0  calOffset=0.0  calMax=inf  calMin=-inf  calFormat='-1'  calUnit=''  calHelp=''  calAccess=1  calFunction=raptor_xcp_function(gcb)  calDispHeaders=off  calColHeaders={'Col1' 'Col2' 'Col3'}  calRowHeaders={'Row1' 'Row2' 'Row3'}
      settings: SourceProductName=Raptor
  raptor_adjustment2 : Raptor_lib/Data Storage/raptor_adjustment  paramName='Cal_EAU_On_DelayTime'  nameSource=Parameter  initValue=0.00  dataType=double  storage=Calibration  calDispType=Number  calEnum={'False', 'True'}  calGain=1.0  calOffset=0.0  calMax=inf  calMin=-inf  calFormat='-1'  calUnit=''  calHelp=''  calAccess=1  calFunction=raptor_xcp_function(gcb)  calDispHeaders=off  calColHeaders={'Col1' 'Col2' 'Col3'}  calRowHeaders={'Row1' 'Row2' 'Row3'}
      settings: SourceProductName=Raptor
  raptor_adjustment3 : Raptor_lib/Data Storage/raptor_adjustment  paramName='Cal_EAU_Off_DelayTime'  nameSource=Parameter  initValue=100  dataType=double  storage=Calibration  calDispType=Number  calEnum={'False', 'True'}  calGain=1.0  calOffset=0.0  calMax=inf  calMin=-inf  calFormat='-1'  calUnit=''  calHelp=''  calAccess=1  calFunction=raptor_xcp_function(gcb)  calDispHeaders=off  calColHeaders={'Col1' 'Col2' 'Col3'}  calRowHeaders={'Row1' 'Row2' 'Row3'}
      settings: SourceProductName=Raptor
  raptor_adjustment6 : Raptor_lib/Data Storage/raptor_adjustment  paramName='Cal_Duty_Low_Saturation'  nameSource=Parameter  initValue=0  dataType=double  storage=Calibration  calDispType=Number  calEnum={'False', 'True'}  calGain=1.0  calOffset=0.0  calMax=inf  calMin=-inf  calFormat='-1'  calUnit=''  calHelp=''  calAccess=1  calFunction=raptor_xcp_function(gcb)  calDispHeaders=off  calColHeaders={'Col1' 'Col2' 'Col3'}  calRowHeaders={'Row1' 'Row2' 'Row3'}
      settings: SourceProductName=Raptor
  raptor_adjustment7 : Raptor_lib/Data Storage/raptor_adjustment  paramName='Cal_Duty_Up_Saturation'  nameSource=Parameter  initValue=100  dataType=double  storage=Calibration  calDispType=Number  calEnum={'False', 'True'}  calGain=1.0  calOffset=0.0  calMax=inf  calMin=-inf  calFormat='-1'  calUnit=''  calHelp=''  calAccess=1  calFunction=raptor_xcp_function(gcb)  calDispHeaders=off  calColHeaders={'Col1' 'Col2' 'Col3'}  calRowHeaders={'Row1' 'Row2' 'Row3'}
      settings: SourceProductName=Raptor
  raptor_adjustment8 : Raptor_lib/Data Storage/raptor_adjustment  paramName='Cal_Cooling_Water_Temp_LimitLow'  nameSource=Parameter  initValue=50  dataType=double  storage=Calibration  calDispType=Number  calEnum={'False', 'True'}  calGain=1.0  calOffset=0.0  calMax=inf  calMin=-inf  calFormat='-1'  calUnit=''  calHelp=''  calAccess=1  calFunction=raptor_xcp_function(gcb)  calDispHeaders=off  calColHeaders={'Col1' 'Col2' 'Col3'}  calRowHeaders={'Row1' 'Row2' 'Row3'}
      settings: SourceProductName=Raptor
  raptor_data_read1 : Raptor_lib/Data Storage/raptor_data_read  dataName='EPT_BPOBU_CURR'  dataShape=Scalar  idxSource=Input  idxRow=1  idxCol=1
      settings: SourceProductName=Raptor
  raptor_data_read2 : Raptor_lib/Data Storage/raptor_data_read  dataName='Relay_DCDC_12V'  dataShape=Scalar  idxSource=Input  idxRow=1  idxCol=1
      settings: SourceProductName=Raptor
  raptor_data_read3 : Raptor_lib/Data Storage/raptor_data_read  dataName='A105_Cooling_Oil_Temp_in'  dataShape=Scalar  idxSource=Input  idxRow=1  idxCol=1
      settings: SourceProductName=Raptor
  raptor_data_read4 : Raptor_lib/Data Storage/raptor_data_read  dataName='EPT_BPOBU_VOLT'  dataShape=Scalar  idxSource=Input  idxRow=1  idxCol=1
      settings: SourceProductName=Raptor
  raptor_data_read6 : Raptor_lib/Data Storage/raptor_data_read  dataName='K37_LSD_Relay_EAU1'  dataShape=Scalar  idxSource=Input  idxRow=1  idxCol=1
      settings: SourceProductName=Raptor
  raptor_data_read7 : Raptor_lib/Data Storage/raptor_data_read  dataName='A17_Cooling_Water_Temp_in'  dataShape=Scalar  idxSource=Input  idxRow=1  idxCol=1
      settings: SourceProductName=Raptor
  raptor_data_read8 : Raptor_lib/Data Storage/raptor_data_read  dataName='K19_LSD_Relay_EAU2'  dataShape=Scalar  idxSource=Input  idxRow=1  idxCol=1
      settings: SourceProductName=Raptor
  raptor_data_read9 : Raptor_lib/Data Storage/raptor_data_read  dataName='Max_CellT'  dataShape=Scalar  idxSource=Input  idxRow=1  idxCol=1
      settings: SourceProductName=Raptor
  raptor_data_write1 : Raptor_lib/Data Storage/raptor_data_write  dataName='K55_LSD_Relay_WC'  dataShape=Scalar  idxSource=Input Port  idxRow=1  idxCol=1
      settings: SourceProductName=Raptor
  raptor_data_write2 : Raptor_lib/Data Storage/raptor_data_write  dataName='A23_LSD_PWM_Duty'  dataShape=Scalar  idxSource=Input Port  idxRow=1  idxCol=1
      settings: SourceProductName=Raptor
  raptor_data_write3 : Raptor_lib/Data Storage/raptor_data_write  dataName='A93_LSD_PWM_Duty'  dataShape=Scalar  idxSource=Input Port  idxRow=1  idxCol=1
      settings: SourceProductName=Raptor
  raptor_data_write4 : Raptor_lib/Data Storage/raptor_data_write  dataName='A46_LSD_Relay_OC'  dataShape=Scalar  idxSource=Input Port  idxRow=1  idxCol=1
      settings: SourceProductName=Raptor
  raptor_data_write5 : Raptor_lib/Data Storage/raptor_data_write  dataName='K37_LSD_Relay_EAU1'  dataShape=Scalar  idxSource=Input Port  idxRow=1  idxCol=1
      settings: SourceProductName=Raptor
  raptor_data_write6 : Raptor_lib/Data Storage/raptor_data_write  dataName='K88_LSD_PWM_Duty'  dataShape=Scalar  idxSource=Input Port  idxRow=1  idxCol=1
      settings: SourceProductName=Raptor
  raptor_measurement2 : Raptor_lib/Data Storage/raptor_measurement  paramName='Oil_Temp'  nameSource=Parameter  calDispType=Number  calEnum={'False', 'True'}  calGain=1.0  calOffset=0.0  calMax=inf  calMin=-inf  calFormat='-1'  calUnit=''  calHelp=''  calAccess=1  calFunction=raptor_xcp_function(gcb)  calVisible=on
      settings: SourceProductName=Raptor
  raptor_measurement3 : Raptor_lib/Data Storage/raptor_measurement  paramName='Water_Temp'  nameSource=Parameter  calDispType=Number  calEnum={'False', 'True'}  calGain=1.0  calOffset=0.0  calMax=inf  calMin=-inf  calFormat='-1'  calUnit=''  calHelp=''  calAccess=1  calFunction=raptor_xcp_function(gcb)  calVisible=on
      settings: SourceProductName=Raptor
  raptor_override1 : Raptor_lib/Data Storage/raptor_override  paramName='Cal_Motor_Cooling_System_Output'  nameSource=Parameter  measurement=None  calDispType=Number  calEnum={'False', 'True'}  calGain=1.0  calOffset=0.0  calMax=inf  calMin=-inf  calFormat='-1'  calUnit=''  calHelp=''  calAccess=1  calFunction=[raptor_xcp_function(gcb) '|' raptor_get_param_eval(gcb, 'paramName') '_Override']
      settings: SourceProductName=Raptor
  raptor_override2 : Raptor_lib/Data Storage/raptor_override  paramName='Cal_A23_Duty'  nameSource=Parameter  measurement=None  calDispType=Number  calEnum={'False', 'True'}  calGain=1.0  calOffset=0.0  calMax=inf  calMin=-inf  calFormat='-1'  calUnit=''  calHelp=''  calAccess=1  calFunction=[raptor_xcp_function(gcb) '|' raptor_get_param_eval(gcb, 'paramName') '_Override']
      settings: SourceProductName=Raptor
  raptor_override3 : Raptor_lib/Data Storage/raptor_override  paramName='Cal_Water_Temp'  nameSource=Parameter  measurement=None  calDispType=Number  calEnum={'False', 'True'}  calGain=1.0  calOffset=0.0  calMax=inf  calMin=-inf  calFormat='-1'  calUnit=''  calHelp=''  calAccess=1  calFunction=[raptor_xcp_function(gcb) '|' raptor_get_param_eval(gcb, 'paramName') '_Override']
      settings: SourceProductName=Raptor
  raptor_override4 : Raptor_lib/Data Storage/raptor_override  paramName='Cal_A93_Duty'  nameSource=Parameter  measurement=None  calDispType=Number  calEnum={'False', 'True'}  calGain=1.0  calOffset=0.0  calMax=inf  calMin=-inf  calFormat='-1'  calUnit=''  calHelp=''  calAccess=1  calFunction=[raptor_xcp_function(gcb) '|' raptor_get_param_eval(gcb, 'paramName') '_Override']
      settings: SourceProductName=Raptor
  raptor_override5 : Raptor_lib/Data Storage/raptor_override  paramName='Cal_Oil_Temp'  nameSource=Parameter  measurement=None  calDispType=Number  calEnum={'False', 'True'}  calGain=1.0  calOffset=0.0  calMax=inf  calMin=-inf  calFormat='-1'  calUnit=''  calHelp=''  calAccess=1  calFunction=[raptor_xcp_function(gcb) '|' raptor_get_param_eval(gcb, 'paramName') '_Override']
      settings: SourceProductName=Raptor
  raptor_override6 : Raptor_lib/Data Storage/raptor_override  paramName='Cal_K88_Duty'  nameSource=Parameter  measurement=None  calDispType=Number  calEnum={'False', 'True'}  calGain=1.0  calOffset=0.0  calMax=inf  calMin=-inf  calFormat='-1'  calUnit=''  calHelp=''  calAccess=1  calFunction=[raptor_xcp_function(gcb) '|' raptor_get_param_eval(gcb, 'paramName') '_Override']
      settings: SourceProductName=Raptor
  raptor_override7 : Raptor_lib/Data Storage/raptor_override  paramName='Cal_OBU_Cooling_System_Output'  nameSource=Parameter  measurement=None  calDispType=Number  calEnum={'False', 'True'}  calGain=1.0  calOffset=0.0  calMax=inf  calMin=-inf  calFormat='-1'  calUnit=''  calHelp=''  calAccess=1  calFunction=[raptor_xcp_function(gcb) '|' raptor_get_param_eval(gcb, 'paramName') '_Override']
      settings: SourceProductName=Raptor
  raptor_table_1d1 : Raptor_lib/Table Lookup/raptor_table_1d  dataName='CoolingSystemTemp2Ft'  initValue=[0.5,1,5,8,10]  dataType=double  storage=Calibration  initValueX=[0,35,40,45,55]  dataTypeXY=double  storageXY=Calibration  calVisible=on  showTable=on  calGain=1.0  calOffset=0.0  calMax=Inf  calMin=-Inf  calFormat='-1'  calUnit=''  calHelp=''  showBreakpoint=on  dataNameX=[]  calGainX=1.0  calOffsetX=0.0  calMaxX=Inf  calMinX=-Inf  calFormatX='-1'  calUnitX=''  calHelpX=''  calAccess=1  calFunction=raptor_xcp_function(gcb)  measureEnable=off  mName=[raptor_get_param_eval(gcb,'dataName'), '_Output']
      settings: SourceProductName=Raptor
  raptor_table_1d2 : Raptor_lib/Table Lookup/raptor_table_1d  dataName='PW2PumpDuty'  initValue=|  dataType=double  storage=Calibration  initValueX=|  dataTypeXY=double  storageXY=Calibration  calVisible=on  showTable=on  calGain=1.0  calOffset=0.0  calMax=Inf  calMin=-Inf  calFormat='-1'  calUnit=''  calHelp=''  showBreakpoint=on  dataNameX=[]  calGainX=1.0  calOffsetX=0.0  calMaxX=Inf  calMinX=-Inf  calFormatX='-1'  calUnitX=''  calHelpX=''  calAccess=1  calFunction=raptor_xcp_function(gcb)  measureEnable=off  mName=[raptor_get_param_eval(gcb,'dataName'), '_Output']
      initValue=|
      | [10
      | 10
      | 20
      | 30
      | 40
      | 50
      | 60
      | 80
      | 100
      | 100
      | 100
      | ]
      initValueX=|
      | [0
      | 2.5
      | 5
      | 7.5
      | 10
      | 12.5
      | 15
      | 17.5
      | 20
      | 22.5
      | 25
      | ]
      settings: SourceProductName=Raptor
  raptor_table_1d3 : Raptor_lib/Table Lookup/raptor_table_1d  dataName='Tcell2BlowerDuty'  initValue="[30\t40\t50\t55]"  dataType=double  storage=Calibration  initValueX="[60\t70\t100\t100]"  dataTypeXY=double  storageXY=Calibration  calVisible=on  showTable=on  calGain=1.0  calOffset=0.0  calMax=Inf  calMin=-Inf  calFormat='-1'  calUnit=''  calHelp=''  showBreakpoint=on  dataNameX=[]  calGainX=1.0  calOffsetX=0.0  calMaxX=Inf  calMinX=-Inf  calFormatX='-1'  calUnitX=''  calHelpX=''  calAccess=1  calFunction=raptor_xcp_function(gcb)  measureEnable=off  mName=[raptor_get_param_eval(gcb,'dataName'), '_Output']
      settings: SourceProductName=Raptor
  raptor_table_1d7 : Raptor_lib/Table Lookup/raptor_table_1d  dataName='KY_Part_ADC2Degree'  initValue=|  dataType=double  storage=Calibration  initValueX=|  dataTypeXY=double  storageXY=Calibration  calVisible=on  showTable=on  calGain=1.0  calOffset=0.0  calMax=Inf  calMin=-Inf  calFormat='-1'  calUnit=''  calHelp=''  showBreakpoint=on  dataNameX=[]  calGainX=1.0  calOffsetX=0.0  calMaxX=Inf  calMinX=-Inf  calFormatX='-1'  calUnitX=''  calHelpX=''  calAccess=1  calFunction=raptor_xcp_function(gcb)  measureEnable=off  mName=[raptor_get_param_eval(gcb,'dataName'), '_Output']
      initValue=|
      | [0
      | 5
      | 10
      | 15
      | 20
      | 25
      | 30
      | 35
      | 40
      | 45
      | 50
      | 55
      | 60
      | 65
      | 70
      | 75
      | 80
      | 85
      | 90
      | 95
      | 100
      | 105
      | 110
      | 115
      | 120
      | 125
      | ]
      initValueX=|
      | [ 4.73 
      |  4.67 
      |  4.58 
      |  4.47 
      |  4.34 
      |  4.20 
      |  4.04 
      |  3.85 
      |  3.67 
      |  3.47 
      |  3.25 
      |  3.04 
      |  2.81 
      |  2.58 
      |  2.38 
      |  2.17 
      |  1.96 
      |  1.77 
      |  1.61 
      |  1.45 
      |  1.32 
      |  1.23 
      |  1.07 
      |  0.99 
      |  0.90 
      |  0.86 
      | ]
      settings: SourceProductName=Raptor
  wires:
  raptor_table_1d2/1 -> Saturation Dynamic3/2
  raptor_table_1d1/1 -> Product1/1, Product/1
  raptor_adjustment6/1 -> Saturation Dynamic3/3
  Saturation Dynamic1/1 -> Demux3/1
  Data Type Conversion5/1 -> raptor_data_write6/1
  raptor_adjustment1/1 -> Relational Operator4/2
  Subtract1/1 -> Data Type Conversion1/1
  Demux/2 -> Subtract1/2
  Latch1/1(Output) -> Mux/4
  Data Type Conversion1/1 -> raptor_data_write2/1
  Gain4/1 -> Data Type Conversion2/1
  raptor_adjustment13/1 -> Delay5/2(TimeCount)
  raptor_table_1d3/1 -> raptor_override6/1
  NOT/1 -> Delay3/1(Condition)
  Delay5/1(Output) -> Latch/1(Latch)
  Delay3/1(Output) -> Latch2/2(Reset)
  raptor_adjustment8/1 -> Relational Operator5/2
  Demux/1 -> Data Type Conversion/1
  raptor_adjustment15/1 -> Relational Operator6/2
  Product2/1 -> Gain/1
  raptor_data_read6/1 -> raptor_override1/1
  raptor_override1/1 -> Switch/2
  Delay6/1(Output) -> Latch1/2(Reset)
  Switch/1 -> Demux/1
  Delay1/1(Output) -> Latch2/1(Latch)
  raptor_adjustment12/1 -> Delay2/2(TimeCount)
  Demux/4 -> Data Type Conversion4/1
  Product1/1 -> raptor_override4/1
  Demux/3 -> Data Type Conversion3/1
  Data Type Conversion4/1 -> raptor_data_write4/1
  Mux/1 -> Switch/1
  raptor_adjustment14/1 -> Delay7/2(TimeCount)
  Latch/1(Output) -> Mux/1
  raptor_override3/1 -> Mux1/1, Relational Operator5/1, Relational Operator4/1
  Relational Operator7/1 -> Delay6/1(Condition)
  raptor_table_1d7/1 -> Demux2/1
  Relational Operator5/1 -> Delay2/1(Condition)
  raptor_data_read3/1 -> Mux2/2
  Data Type Conversion2/1 -> raptor_table_1d7/1
  raptor_override5/1 -> Relational Operator6/1, Relational Operator7/1, Mux1/2
  Mux2/1 -> Gain4/1
  raptor_data_read7/1 -> Mux2/1
  Demux2/2 -> raptor_override5/1, raptor_measurement2/1
  Mux1/1 -> raptor_table_1d1/1
  Demux2/1 -> raptor_override3/1, raptor_measurement3/1
  Data Type Conversion/1 -> raptor_data_write1/1
  Delay7/1(Output) -> Latch1/1(Latch)
  raptor_adjustment3/1 -> Delay3/2(TimeCount)
  raptor_data_read9/1 -> raptor_table_1d3/1
  raptor_data_read2/1 -> Delay1/1(Condition), NOT/1
  raptor_adjustment2/1 -> Delay1/2(TimeCount)
  Delay2/1(Output) -> Latch/2(Reset)
  raptor_adjustment16/1 -> Relational Operator7/2
  Latch2/1(Output) -> raptor_data_write5/1
  Gain/1 -> raptor_table_1d2/1
  Product/1 -> raptor_override2/1
  raptor_override7/1 -> Switch1/2
  Subtract2/1 -> Data Type Conversion5/1
  raptor_data_read8/1 -> raptor_override7/1
  Data Type Conversion3/1 -> raptor_data_write3/1
  raptor_override6/1 -> Switch1/1
  Relational Operator4/1 -> Delay5/1(Condition)
  Relational Operator6/1 -> Delay7/1(Condition)
  raptor_override2/1 -> Mux3/1
  raptor_data_read1/1 -> Product2/1
  Demux3/1 -> Mux/2
  raptor_adjustment7/1 -> Saturation Dynamic3/1, Subtract2/1, Subtract1/1, Saturation Dynamic1/1
  raptor_adjustment17/1 -> Delay6/2(TimeCount)
  Demux3/2 -> Mux/3
  Saturation Dynamic3/1 -> Product1/2, Product/2
  Mux3/1 -> Saturation Dynamic1/2
  raptor_data_read4/1 -> Product2/2
  raptor_override4/1 -> Mux3/2
  Switch1/1 -> Subtract2/2

== system EPT/Foreground_TimeBase_5ms/Oil//Water//Pack Cooling System/Delay1 ==
  Condition : Inport
  TimeCount : Inport  Port=2
  Constant10 : Constant
  Constant11 : Constant  Value=0
  Constant8 : Constant  Value=0
  CycleTrigger : Subsystem
  Switch2 : Switch  Threshold=1
  Switch3 : Switch  Threshold=1
  Unit Delay1 : UnitDelay  SampleTime=-1  HasFrameUpgradeWarning=on
  Unit Delay3 : UnitDelay  SampleTime=-1  HasFrameUpgradeWarning=on
  Output : Outport  VectorParamsAs1DForOutWhenUnconnected=off
  wires:
  TimeCount/1 -> CycleTrigger/2(In2)
  Condition/1 -> Switch3/2
  Constant8/1 -> Switch2/1
  CycleTrigger/1(Trigger) -> Switch2/2, Unit Delay3/1
  Constant10/1 -> Switch2/3
  Switch3/1 -> CycleTrigger/1(In1)
  Switch2/1 -> Unit Delay1/1
  Constant11/1 -> Switch3/3
  Unit Delay1/1 -> Switch3/1
  Unit Delay3/1 -> Output/1
